simulink subsystem "BEVController_refsub_Basic"  (R2023a)
settings: Solver=VariableStepAuto  StartTime=0.0  StopTime=10.0  RelTol=1e-3
undefined symbols (not defined in the file): bevControl, motorDriveUnit
settings Model: Creator=isaacito  LastModifiedBy=antaeug
settings OptimizationCC: ReuseModelBlockBuffer=off

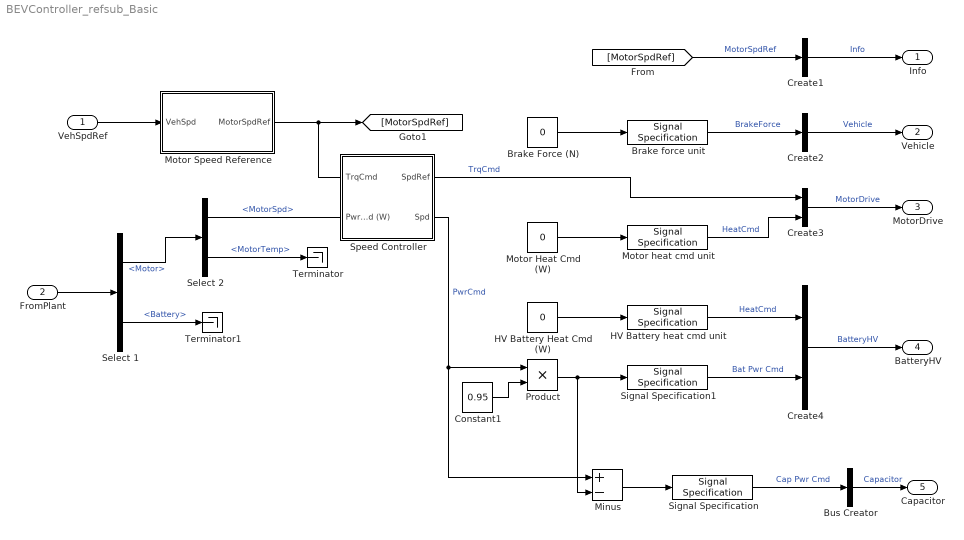
== system BEVController_refsub_Basic ==
  VehSpdRef : Inport
  FromPlant : Inport  Port=2
  Brake Force (N) : Constant  Value=0
  Brake force unit : SignalSpecification  Unit=N
  Bus Creator : BusCreator  Inputs=1
  Constant1 : Constant  Value=0.95
  Create1 : BusCreator  Inputs=1
  Create2 : BusCreator  Inputs=1
  Create3 : BusCreator  Inputs=2
  Create4 : BusCreator  Inputs=2
  HV Battery Heat Cmd (W) : Constant  Value=0
  HV Battery heat cmd unit : SignalSpecification  Unit=W
  Minus : Sum  Inputs=+-
  Motor Heat Cmd (W) : Constant  Value=0
  Motor Speed Reference : Subsystem
  Motor heat cmd unit : SignalSpecification  Unit=W
  Product : Product
  Select 1 : BusSelector  OutputSignals=Motor,Battery
  Select 2 : BusSelector  OutputSignals=MotorSpd,MotorTemp
  Signal Specification : SignalSpecification  Unit=W
  Signal Specification1 : SignalSpecification  Unit=W
  Speed Controller : Subsystem
  Terminator : Terminator
  Terminator1 : Terminator
  Info : Outport
  Vehicle : Outport  Port=2
  MotorDrive : Outport  Port=3
  BatteryHV : Outport  Port=4
  Capacitor : Outport  Port=5
  wires:
  Motor Speed Reference/1(MotorSpdRef) -> [MotorSpdRef], Speed Controller/1(SpdRef)
  Select 2/1 -> Speed Controller/2(Spd)  "<MotorSpd>"
  Speed Controller/1(TrqCmd) -> Create3/1  "TrqCmd"
  VehSpdRef/1 -> Motor Speed Reference/1(VehSpd)
  Brake Force (N)/1 -> Brake force unit/1
  FromPlant/1 -> Select 1/1
  Select 1/1 -> Select 2/1  "<Motor>"
  [MotorSpdRef] -> Create1/1  "MotorSpdRef"
  Create1/1 -> Info/1  "Info"
  Create2/1 -> Vehicle/1  "Vehicle"
  Create3/1 -> MotorDrive/1  "MotorDrive"
  Create4/1 -> BatteryHV/1  "BatteryHV"
  Select 1/2 -> Terminator1/1  "<Battery>"
  Motor Heat Cmd (W)/1 -> Motor heat cmd unit/1
  HV Battery Heat Cmd (W)/1 -> HV Battery heat cmd unit/1
  Select 2/2 -> Terminator/1  "<MotorTemp>"
  Motor heat cmd unit/1 -> Create3/2  "HeatCmd"
  HV Battery heat cmd unit/1 -> Create4/1  "HeatCmd"
  Brake force unit/1 -> Create2/1  "BrakeForce"
  Bus Creator/1 -> Capacitor/1  "Capacitor"
  Speed Controller/2(PwrCmd (W)) -> Minus/1, Product/1  "PwrCmd"
  Constant1/1 -> Product/2
  Product/1 -> Minus/2, Signal Specification1/1
  Minus/1 -> Signal Specification/1
  Signal Specification/1 -> Bus Creator/1  "Cap Pwr Cmd"
  Signal Specification1/1 -> Create4/2  "Bat Pwr Cmd"

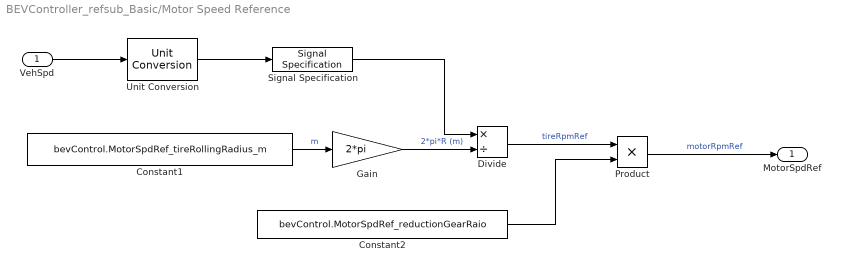
== system BEVController_refsub_Basic/Motor Speed Reference ==
  VehSpd : Inport  Unit=km/hr
  Constant1 : Constant  Value=bevControl.MotorSpdRef_tireRollingRadius_m
  Constant2 : Constant  Value=bevControl.MotorSpdRef_reductionGearRaio
  Divide : Product  Inputs=*/
  Gain : Gain  Gain=2*pi
  Product : Product
  Signal Specification : SignalSpecification  Unit=m/min
  Unit Conversion : UnitConversion
  MotorSpdRef : Outport  Unit=rpm  VectorParamsAs1DForOutWhenUnconnected=off
  wires:
  Constant1/1 -> Gain/1  "m"
  Product/1 -> MotorSpdRef/1  "motorRpmRef"
  Constant2/1 -> Product/2
  Divide/1 -> Product/1  "tireRpmRef"
  Gain/1 -> Divide/2  "2*pi*R (m)"
  Signal Specification/1 -> Divide/1
  Unit Conversion/1 -> Signal Specification/1
  VehSpd/1 -> Unit Conversion/1

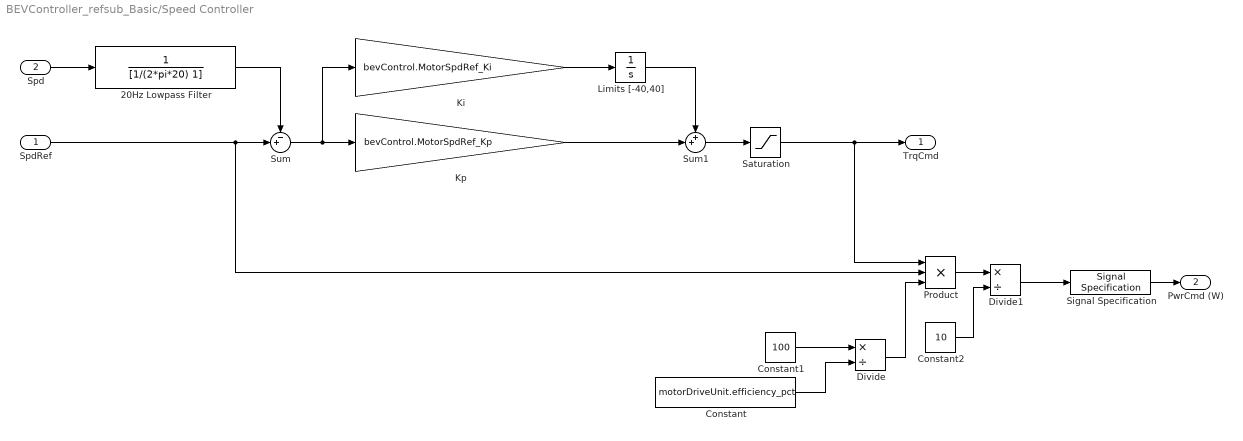
== system BEVController_refsub_Basic/Speed Controller ==
  SpdRef : Inport  Unit=rpm
      settings: AttributesFormatString=%<Unit>
  Spd : Inport  Port=2  Unit=rpm
      settings: AttributesFormatString=%<Unit>
  20Hz Lowpass Filter : TransferFcn  Denominator=[1/(2*pi*20) 1]
  Constant : Constant  Value=motorDriveUnit.efficiency_pct
  Constant1 : Constant  Value=100
  Constant2 : Constant  Value=10
  Divide : Product  Inputs=*/
  Divide1 : Product  Inputs=*/
  Ki : Gain  Gain=bevControl.MotorSpdRef_Ki
  Kp : Gain  Gain=bevControl.MotorSpdRef_Kp
  Limits [-40,40] : Integrator  LimitOutput=on  UpperSaturationLimit=40  LowerSaturationLimit=-40
  Product : Product  Inputs=3
  Saturation : Saturate  UpperLimit=bevControl.MotorDriveUnit_trqMax_Nm  LowerLimit=-bevControl.MotorDriveUnit_trqMax_Nm
      settings: AttributesFormatString=|
      | %<UpperLimit>
      | %<LowerLimit>
  Signal Specification : SignalSpecification  Unit=W
  Sum : Sum  Inputs=-+|
  Sum1 : Sum  Inputs=++|
  TrqCmd : Outport  Unit=N*m  VectorParamsAs1DForOutWhenUnconnected=off
      settings: AttributesFormatString=%<Unit>
  PwrCmd (W) : Outport  Port=2
  wires:
  Constant2/1 -> Divide1/2
  Divide1/1 -> Signal Specification/1
  Product/1 -> Divide1/1
  Divide/1 -> Product/3
  Constant/1 -> Divide/2
  Constant1/1 -> Divide/1
  Signal Specification/1 -> PwrCmd (W)/1
  SpdRef/1 -> Sum/2, Product/2
  Spd/1 -> 20Hz Lowpass Filter/1
  Sum1/1 -> Saturation/1
  Sum/1 -> Ki/1, Kp/1
  Ki/1 -> Limits [-40,40]/1
  Kp/1 -> Sum1/2
  Limits [-40,40]/1 -> Sum1/1
  20Hz Lowpass Filter/1 -> Sum/1
  Saturation/1 -> TrqCmd/1, Product/1
